simulink model "problem4"  (R2019a)
settings: Solver=VariableStepAuto  StartTime=0.0  StopTime=10000  RelTol=1e-3
undefined symbols (not defined in the file): m, n
settings Model: Creator=Avery Peiffer  LastModifiedBy=Avery Peiffer

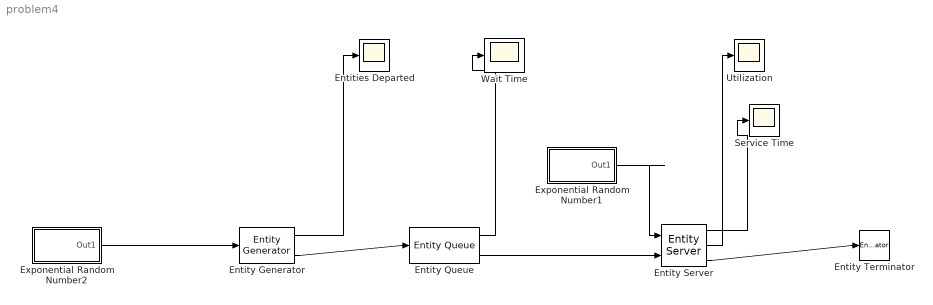
== system problem4 ==
  Entities Departed : Scope
  "Entity Generator " : EntityGenerator  OutputPortMessageModes=n,m  TimeSource=Signal port  Period=2  IntergenerationTimeAction=|  NumberEntitiesDeparted=on  EntityType=Structured  EntityTypeName=Entity
      | dt = rand(1,1);
      | persistent rngInit;
      | if isempty(rngInit)
      |     seed = 12345;
      |     rng(seed);
      |     rngInit = true;
      | end
      | 
      | % Pattern: Exponential distribution
      | mu = 1;
      | x = -mu * log(1 - rand());
      settings: InputPortMap=u1  OutputPortMap=o0,o3
  Entity Queue : EntityQueue  InputPortMessageModes=m  OutputPortMessageModes=n,m  Capacity=1  AverageWait=on
      settings: OutputPortMap=o2,o5
  Entity Server : EntityServer  InputPortMessageModes=n,m  OutputPortMessageModes=n,n,m  Capacity=1  ServiceTimeSource=Signal port  ServiceTimeValue=0.67  ServiceTimeAction=|  AverageWait=on  Utilization=on
      | dt = rand(1,1);
      | persistent rngInit;
      | if isempty(rngInit)
      |     seed = 123;
      |     rng(seed);
      |     rngInit = true;
      | end
      | 
      | % Pattern: Exponential distribution
      | mu = 0.67;
      | x = -mu * log(1 - rand());
      settings: InputPortMap=u0,u2  OutputPortMap=o4,o5,o9
  Entity Terminator : EntityTerminator  InputPortMessageModes=m
  Exponential Random Number1 : Subsystem  mask(Exponential Random Number){mean=0.67, seed=100}
      mask prompts: seed "Random Seed"
      mask help: This block generate a random number with exponential distribution.
      mask Display: disp(['mean=' num2str(mean,2)],"texmode","on");
  Exponential Random Number2 : Subsystem  mask(Exponential Random Number){mean=1, seed=24}
      mask prompts: seed "Random Seed"
      mask help: This block generate a random number with exponential distribution.
      mask Display: disp(['mean=' num2str(mean,2)],"texmode","on");
  Service Time : Scope
  Utilization : Scope
  Wait Time : Scope
  wires:
  Entity Queue/1 -> Wait Time/1
  "Entity Generator "/2 -> Entity Queue/1
  Entity Queue/2 -> Entity Server/2
  Entity Server/3 -> Entity Terminator/1
  "Entity Generator "/1 -> Entities Departed/1
  Entity Server/2 -> Utilization/1
  Entity Server/1 -> Service Time/1
  Exponential Random Number2/1(Out1) -> "Entity Generator "/1
  Exponential Random Number1/1(Out1) -> Entity Server/1

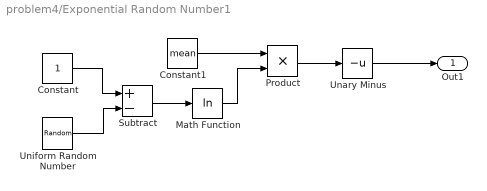
== system problem4/Exponential Random Number1 ==
  Constant : Constant
  Constant1 : Constant  Value=mean
  Math Function : Math  Operator=log  SaturateOnIntegerOverflow=on
  Product : Product  RndMeth=Zero
  Subtract : Sum  Inputs=+-
  Unary Minus : UnaryMinus
  Uniform Random Number : UniformRandomNumber  Minimum=0  Seed=seed
  Out1 : Outport  VectorParamsAs1DForOutWhenUnconnected=on
  wires:
  Subtract/1 -> Math Function/1
  Math Function/1 -> Product/2
  Unary Minus/1 -> Out1/1
  Product/1 -> Unary Minus/1
  Constant/1 -> Subtract/1
  Uniform Random Number/1 -> Subtract/2
  Constant1/1 -> Product/1

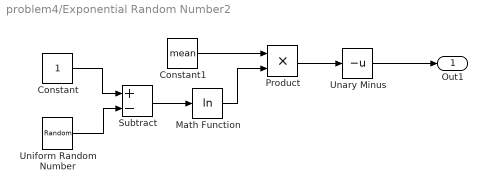
== system problem4/Exponential Random Number2 ==
  Constant : Constant
  Constant1 : Constant  Value=mean
  Math Function : Math  Operator=log  SaturateOnIntegerOverflow=on
  Product : Product  RndMeth=Zero
  Subtract : Sum  Inputs=+-
  Unary Minus : UnaryMinus
  Uniform Random Number : UniformRandomNumber  Minimum=0  Seed=seed
  Out1 : Outport  VectorParamsAs1DForOutWhenUnconnected=on
  wires:
  Subtract/1 -> Math Function/1
  Math Function/1 -> Product/2
  Unary Minus/1 -> Out1/1
  Product/1 -> Unary Minus/1
  Constant/1 -> Subtract/1
  Uniform Random Number/1 -> Subtract/2
  Constant1/1 -> Product/1
